simulink model "CombinedModel_KellenHassel"  (R2025b)
settings: Solver=VariableStepAuto  StartTime=0.0  StopTime=10.0  RelTol=1e-3

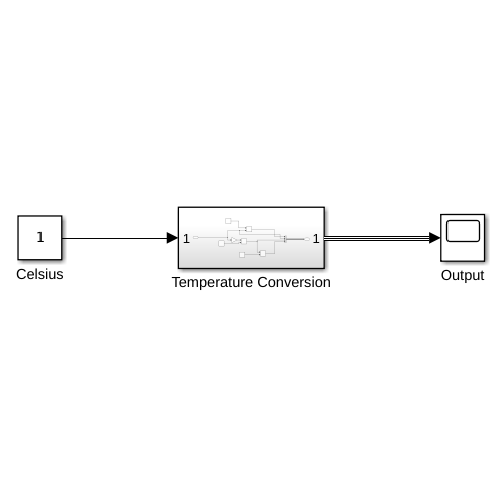
[thumbnail: Simulink's stored preview of the top-level diagram]
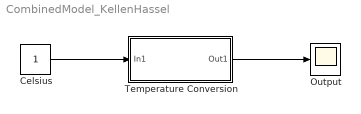
== system CombinedModel_KellenHassel ==
  Celsius : Constant
  Output : Scope
      settings: ActiveDisplayYMinimum=-233.26328995402707  ActiveDisplayYMaximum=592.96951621888866  YLabel=Temperature
  Temperature Conversion : Subsystem
  wires:
  Celsius/1 -> Temperature Conversion/1(In1)
  Temperature Conversion/1(Out1) -> Output/1

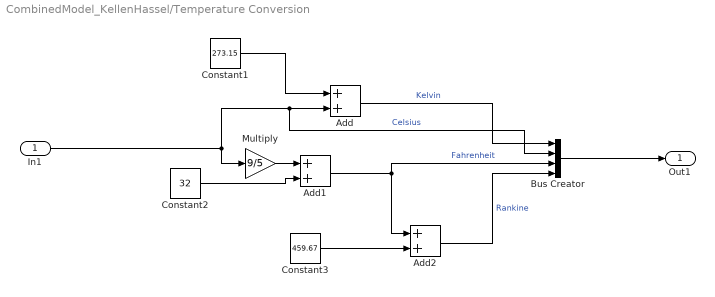
== system CombinedModel_KellenHassel/Temperature Conversion ==
  In1 : Inport
  Add : Sum
  Add1 : Sum
  Add2 : Sum
  Bus Creator : BusCreator  Inputs=4
  Constant1 : Constant  Value=273.15
  Constant2 : Constant  Value=32
  Constant3 : Constant  Value=459.67
  Multiply : Gain  Gain=9/5
  Out1 : Outport
  wires:
  Multiply/1 -> Add1/1
  Constant3/1 -> Add2/2
  In1/1 -> Bus Creator/2, Add/2, Multiply/1  "Celsius"
  Add1/1 -> Bus Creator/3, Add2/1  "Fahrenheit"
  Add2/1 -> Bus Creator/4  "Rankine"
  Constant2/1 -> Add1/2
  Add/1 -> Bus Creator/1  "Kelvin"
  Constant1/1 -> Add/1
  Bus Creator/1 -> Out1/1
